simulink model "ExampleStructToBus"  (R2024a)
settings: Solver=FixedStepAuto  StartTime=0.0  StopTime=0  FixedStep=0.01  RelTol=1e-3
values from neighbouring files (symbols this model uses):
  structExample = struct()    [INIT_ExampleStructToBus.m]
settings Model: Creator=Scythe  LastModifiedBy=damerius
settings SolverCC: ConcurrentTasks=on
settings DataIOCC: SaveOutput=off  SignalLogging=off  DSMLogging=off  SaveTime=off  ReturnWorkspaceOutputs=off
settings OptimizationCC: DefaultParameterBehavior=Inlined  ZeroExternalMemoryAtStartup=off  ZeroInternalMemoryAtStartup=off  SimCompilerOptimization=on
settings DebuggingCC: UnconnectedInputMsg=warning  UnconnectedOutputMsg=warning  UnconnectedLineMsg=warning
settings HardwareCC: ProdBitPerLong=64  ProdHWDeviceType=Intel->x86-64 (Linux 64)
settings ModelReferenceCC: EnableRefExpFcnMdlSchedulingChecks=on
settings SFSimCC: SimParseCustomCode=off  SimGenImportedTypeDefs=on  SimTargetLang=C++
settings RTWCC: GenCodeOnly=on  PackageGeneratedCodeAndArtifacts=on  PackageName=PackNGo  RTWVerbose=off  BuildConfiguration=Faster Runs  TargetLang=C++
settings CodeAppCC: ForceParamTrailComments=on  MaxIdLength=128  StateflowObjectComments=on  MATLABSourceComments=on  UseSimReservedNames=on
settings GRTTargetCC: TargetLangStandard=C++11 (ISO)  MatFileLogging=off  CodeInterfacePackaging=C++ class

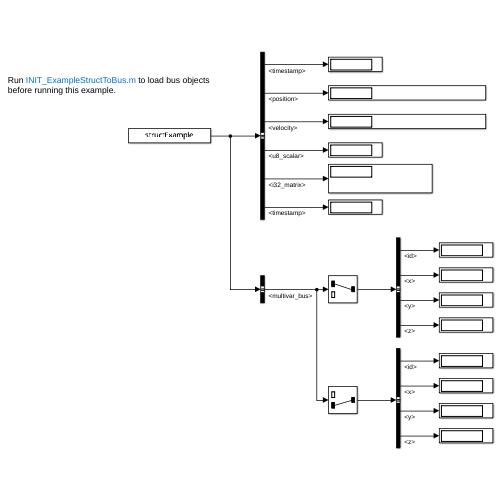
[thumbnail: Simulink's stored preview of the top-level diagram]
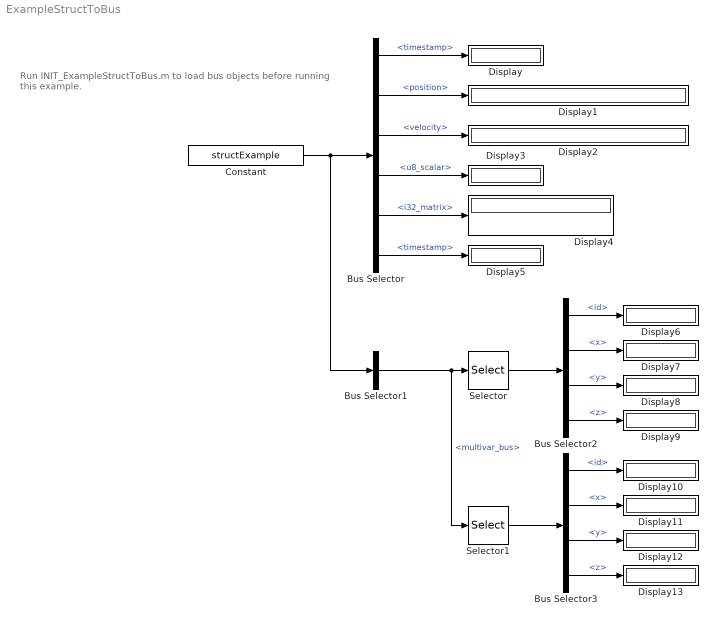
== system ExampleStructToBus ==
  note: Run INIT_ExampleStructToBus.m to load bus objects before running this example.
  Bus Selector : BusSelector  OutputSignals=timestamp,position,velocity,types.u8_scalar,types.i32_matrix,nested_bus.timestamp
  Bus Selector1 : BusSelector  OutputSignals=multivar_bus
  Bus Selector2 : BusSelector  OutputSignals=id,x,y,z
  Bus Selector3 : BusSelector  OutputSignals=id,x,y,z
  Constant : Constant  Value=structExample  OutDataTypeStr=Bus: busExample
  Display{,1..13} (14 alike) : Display
  Selector : Selector  InputPortWidth=2  IndexOptions=Index vector (dialog)  Indices=1  OutputSizes=1
  Selector1 : Selector  InputPortWidth=2  IndexOptions=Index vector (dialog)  Indices=2  OutputSizes=1
  wires:
  Constant/1 -> Bus Selector1/1, Bus Selector/1
  Bus Selector/1 -> Display/1  "<timestamp>"
  Bus Selector/2 -> Display1/1  "<position>"
  Bus Selector/4 -> Display3/1  "<u8_scalar>"
  Bus Selector/3 -> Display2/1  "<velocity>"
  Bus Selector/5 -> Display4/1  "<i32_matrix>"
  Bus Selector/6 -> Display5/1  "<timestamp>"
  Bus Selector1/1 -> Selector1/1, Selector/1  "<multivar_bus>"
  Selector/1 -> Bus Selector2/1
  Bus Selector2/1 -> Display6/1  "<id>"
  Bus Selector2/2 -> Display7/1  "<x>"
  Bus Selector2/3 -> Display8/1  "<y>"
  Bus Selector2/4 -> Display9/1  "<z>"
  Bus Selector3/4 -> Display13/1  "<z>"
  Bus Selector3/3 -> Display12/1  "<y>"
  Bus Selector3/2 -> Display11/1  "<x>"
  Bus Selector3/1 -> Display10/1  "<id>"
  Selector1/1 -> Bus Selector3/1
